simulink model "sampleModel2000"  (R2023a)
settings: Solver=VariableStepAuto  StartTime=0.0  StopTime=10.0  RelTol=1e-3
libraries: hdlsllib x4, simulink x2
settings Model: Creator=user1  LastModifiedBy=user1

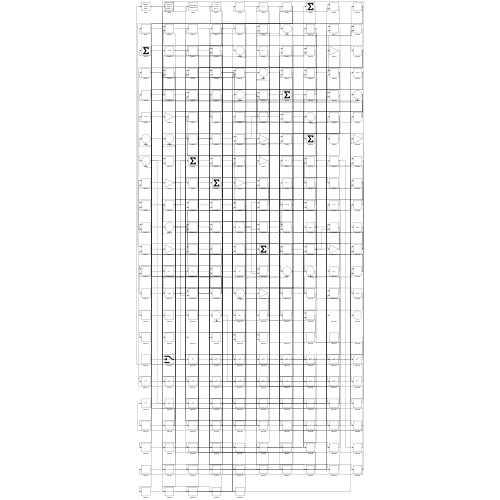
[thumbnail: Simulink's stored preview of the top-level diagram]
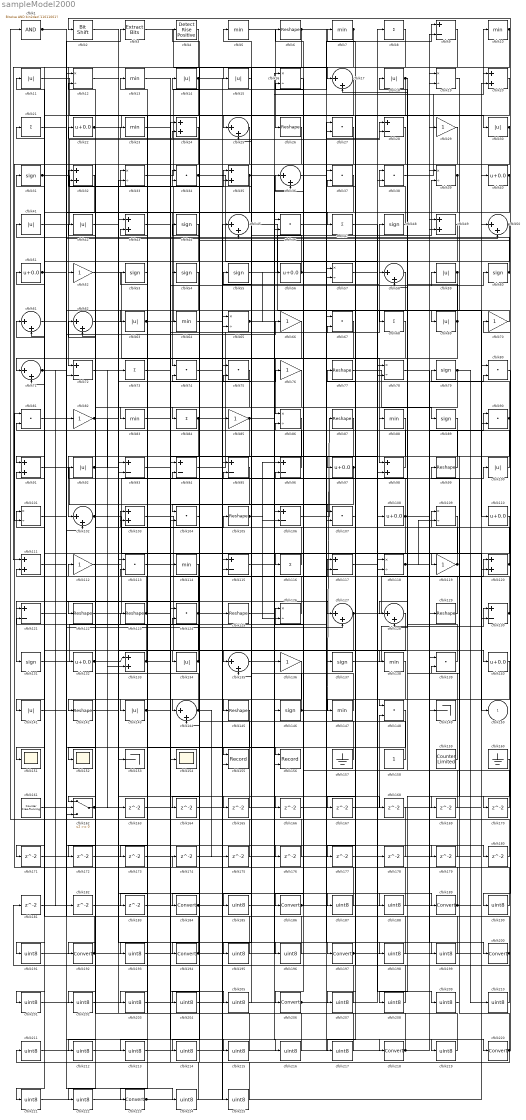
== system sampleModel2000 ==
  cfblk1 : simulink/Logic and Bit Operations/Bitwise Operator  logicop=AND  UseBitMask=on  BitMask=bin2dec('11011001')  BitMaskRealWorld=Stored Integer
      settings: LibrarySourceBlock=|
      | hdlsllib/Logic and Bit
      | Operations/Bitwise
      | Operator
  cfblk{5,7,10,13,23,64,83,88,114,138,147} (11 alike) : MinMax
  cfblk{11,14..15,18,30,41..42,59,63,69,92,100,134,141,143} (15 alike) : Abs  SaturateOnIntegerOverflow=off
  cfblk{12,16,19,33,39,57,65,78,86,101,109,118,126} (13 alike) : Product  Inputs=*/  RndMeth=Zero  SaturateOnIntegerOverflow=on
  cfblk{17,25,36,45,50,58,61..62,71,102,127..128,135,144} (14 alike) : Sum  Inputs=|++
  cfblk{20,24,32,35,43,49,91,98,103,111,120,133} (12 alike) : Sum
  cfblk{27,34,37..38,46,67,74..75,80..81,90,104,107,113,124,139,148} (17 alike) : DotProduct  OutDataTypeStr=Inherit: Inherit via internal rule
  cfblk{6,26,77,87,99,105,122..123,125,129,142,145} (12 alike) : Reshape
  cfblk{9,28,72,93..96,106,115,117,121,130} (12 alike) : Sum  Inputs=+-
  cfblk{22,40,51,56,97,108,110,132,140} (9 alike) : Bias  Bias=0.0  SaturateOnIntegerOverflow=off
  cfblk{29,52,66,70,76,82,85,112,119,136} (10 alike) : Gain
  cfblk{8,21,47,68,73,84,116} (7 alike) : Sum  Inputs=+
  cfblk{31,44,48,53..55,60,79,89,131,137,146} (12 alike) : Signum
  cfblk149 : Terminator
  cfblk151 : Scope
  cfblk152 : Scope
  cfblk153 : Terminator
  cfblk154 : Scope
  cfblk155 : Record  FileSettingsInternal="{\"entries\":[{\"content\":{\"excelSettings\":{\"content\":{},\"type\":\"Streamout.ExcelSettings\"}},\"type\":\"Streamout.FileSettingStorage\",\"uuid\":\"\"}],\"packageUris\":[\"http:\\/\\/schema.mathworks.com\\/mf0\\/streamout_blocks\\/R2020a\"],\"version\":\"1.0\"}"  Layout=[1 1]  SignalsInternal="{\"entries\":[{\"content\":{\"signals\":[{\"content\":{\"blockPath\":[],\"dimensions\":[1],\"domain\":\"\",\"lineColor\":\"#a2142f\",\"plots\":[1],\"port\":1,\"signalID\":5766,\"signalName\":\"XY Graph:1\"},\"type\":\"RecordBlkView.Signal\",\"uuid\":\"\"},{\"content\":{\"blockPath\":[],\"dimensions\":[1],\"domain\":\"\",\"lineColor\":\"#139fff\",\"plots\":[1],\"port\":2,\"signalID\":5769,\"signalName\":\"XY Graph:2\"},\"type\":\"RecordBlkView.Signal\",\"uuid\":\"\"}]},\"type\":\"RecordBlkView.InputSignals\",\"uuid\":\"\"}],\"packageUris\":[\"http:\\/\\/schema.mathworks.com\\/mf0\\/streamout_blocks\\/R2020a\"],\"version\":\"1.0\"}"  VisualizationBindings="{\"xyplotplugin\":{\"info\":[{\"series\":[{\"bindingParametersList\":[{\"parameter\":\"X-Axis\",\"signalID\":5766,\"signalName\":\"XY Graph:1\"},{\"parameter\":\"Y-Axis\",\"signalID\":5769,\"signalName\":\"XY Graph:2\"}],\"seriesID\":56463}],\"subplotID\":1}]}}"  CompatibilityTag=XY  st=-1
  cfblk156 : Record  FileSettingsInternal="{\"entries\":[{\"content\":{\"excelSettings\":{\"content\":{},\"type\":\"Streamout.ExcelSettings\"}},\"type\":\"Streamout.FileSettingStorage\",\"uuid\":\"\"}],\"packageUris\":[\"http:\\/\\/schema.mathworks.com\\/mf0\\/streamout_blocks\\/R2020a\"],\"version\":\"1.0\"}"  Layout=[1 1]  SignalsInternal="{\"entries\":[{\"content\":{\"signals\":[{\"content\":{\"blockPath\":[],\"dimensions\":[1],\"domain\":\"\",\"lineColor\":\"#a2142f\",\"plots\":[1],\"port\":1,\"signalID\":5774,\"signalName\":\"XY Graph:1\"},\"type\":\"RecordBlkView.Signal\",\"uuid\":\"\"},{\"content\":{\"blockPath\":[],\"dimensions\":[1],\"domain\":\"\",\"lineColor\":\"#139fff\",\"plots\":[1],\"port\":2,\"signalID\":5777,\"signalName\":\"XY Graph:2\"},\"type\":\"RecordBlkView.Signal\",\"uuid\":\"\"}]},\"type\":\"RecordBlkView.InputSignals\",\"uuid\":\"\"}],\"packageUris\":[\"http:\\/\\/schema.mathworks.com\\/mf0\\/streamout_blocks\\/R2020a\"],\"version\":\"1.0\"}"  VisualizationBindings="{\"xyplotplugin\":{\"info\":[{\"series\":[{\"bindingParametersList\":[{\"parameter\":\"X-Axis\",\"signalID\":5774,\"signalName\":\"XY Graph:1\"},{\"parameter\":\"Y-Axis\",\"signalID\":5777,\"signalName\":\"XY Graph:2\"}],\"seriesID\":7171}],\"subplotID\":1}]}}"  CompatibilityTag=XY  st=-1
  cfblk157 : Ground
  cfblk158 : Constant  SampleTime=-1
  cfblk159 : hdlsllib/Sources/Counter Limited  uplimit=7  tsamp=-1
  cfblk160 : Ground
  cfblk161 : hdlsllib/Sources/Counter Free-Running  NumBits=16  tsamp=-1
  cfblk162 : Switch  SaturateOnIntegerOverflow=off  InputSameDT=off
  cfblk{163..183} (21 alike) : Delay  SampleTime=1
  cfblk{184,186,189,192,194,197,200,206,218,220,223} (11 alike) : DataTypeConversion  SaturateOnIntegerOverflow=off  RndMeth=Floor
  cfblk{185,187..188,190..191,193,195..196,198..199,201..205,207..217,219,221..222,224..225} (31 alike) : DataTypeConversion  OutDataTypeStr=uint8  SaturateOnIntegerOverflow=off  RndMeth=Floor
  cfblk2 : hdlsllib/Logic and Bit Operations/Bit Shift  mode=Shift Left Logical  N=0
  cfblk3 : simulink/Logic and Bit Operations/Extract Bits  bitsToExtract=Upper half  numBits=8  bitIdxRange=[0 7]  outScalingMode=Preserve fixed-point scaling
      settings: LibrarySourceBlock=|
      | hdlsllib/Logic and Bit
      | Operations/Extract Bits
  cfblk4 : hdlsllib/Logic and Bit Operations/Detect Rise Positive  vinit=0  OutDataTypeStr=boolean
  cfblk150 : Outport  VectorParamsAs1DForOutWhenUnconnected=off
  wires:
  cfblk92/1 -> cfblk73/1, cfblk138/1
  cfblk22/1 -> cfblk25/1, cfblk188/1
  cfblk114/1 -> cfblk131/1
  cfblk105/1 -> cfblk96/1, cfblk106/2, cfblk126/2
  cfblk36/1 -> cfblk189/1
  cfblk162/1 -> cfblk165/1, cfblk166/1
  cfblk88/1 -> cfblk102/1
  cfblk84/1 -> cfblk180/1, cfblk202/1
  cfblk35/1 -> cfblk74/1, cfblk20/1, cfblk117/2
  cfblk77/1 -> cfblk89/1
  cfblk63/1 -> cfblk35/1, cfblk67/2
  cfblk4/1 -> cfblk111/1
  cfblk144/1 -> cfblk4/1, cfblk112/1, cfblk175/1
  cfblk147/1 -> cfblk55/1
  cfblk64/1 -> cfblk60/1
  cfblk54/1 -> cfblk83/1
  cfblk146/1 -> cfblk87/1, cfblk41/1
  cfblk134/1 -> cfblk11/1, cfblk121/2, cfblk123/1
  cfblk38/1 -> cfblk10/1
  cfblk42/1 -> cfblk153/1
  cfblk29/1 -> cfblk184/1
  cfblk124/1 -> cfblk101/1, cfblk58/1, cfblk162/1
  cfblk68/1 -> cfblk86/1
  cfblk16/1 -> cfblk186/1
  cfblk13/1 -> cfblk154/1
  cfblk9/1 -> cfblk14/1
  cfblk87/1 -> cfblk142/1
  cfblk27/1 -> cfblk116/1
  cfblk130/1 -> cfblk33/1, cfblk13/1
  cfblk103/1 -> cfblk135/1
  cfblk52/1 -> cfblk98/1
  cfblk136/1 -> cfblk192/1
  cfblk5/1 -> cfblk26/1
  cfblk102/1 -> cfblk46/1, cfblk150/1, cfblk133/2
  cfblk159/1 -> cfblk18/1
  cfblk98/1 -> cfblk86/2
  cfblk94/1 -> cfblk48/1
  cfblk50/1 -> cfblk122/1, cfblk104/1, cfblk128/1
  cfblk112/1 -> cfblk8/1
  cfblk18/1 -> cfblk88/1, cfblk217/1
  cfblk34/1 -> cfblk118/1, cfblk47/1, cfblk199/1
  cfblk121/1 -> cfblk127/1
  cfblk3/1 -> cfblk17/1
  cfblk59/1 -> cfblk156/1, cfblk162/3
  cfblk143/1 -> cfblk43/2, cfblk168/1
  cfblk110/1 -> cfblk137/1
  cfblk58/1 -> cfblk97/1
  cfblk132/1 -> cfblk133/1, cfblk124/2
  cfblk119/1 -> cfblk109/1, cfblk103/2
  cfblk7/1 -> cfblk72/1, cfblk191/1, cfblk214/1
  cfblk47/1 -> cfblk119/1
  cfblk62/1 -> cfblk125/1
  cfblk123/1 -> cfblk111/2, cfblk205/1
  cfblk100/1 -> cfblk44/1
  cfblk55/1 -> cfblk39/2
  cfblk116/1 -> cfblk5/1
  cfblk158/1 -> cfblk22/1
  cfblk61/1 -> cfblk82/1
  cfblk106/1 -> cfblk40/1
  cfblk122/1 -> cfblk105/1
  cfblk137/1 -> cfblk130/1
  cfblk73/1 -> cfblk59/1
  cfblk141/1 -> cfblk66/1
  cfblk40/1 -> cfblk141/1, cfblk162/2
  cfblk126/1 -> cfblk51/1
  cfblk23/1 -> cfblk218/1
  cfblk41/1 -> cfblk28/1
  cfblk128/1 -> cfblk151/1
  cfblk95/1 -> cfblk194/1
  cfblk45/1 -> cfblk110/1
  cfblk96/1 -> cfblk31/1
  cfblk157/1 -> cfblk126/1
  cfblk25/1 -> cfblk101/2
  cfblk82/1 -> cfblk76/1, cfblk163/1
  cfblk19/1 -> cfblk69/1
  cfblk11/1 -> cfblk93/2
  cfblk133/1 -> cfblk114/1, cfblk81/2, cfblk156/2, cfblk117/1
  cfblk60/1 -> cfblk21/1, cfblk34/2
  cfblk37/1 -> cfblk206/1
  cfblk74/1 -> cfblk85/1
  cfblk69/1 -> cfblk84/1, cfblk17/2
  cfblk120/1 -> cfblk2/1, cfblk77/1, cfblk32/1
  cfblk86/1 -> cfblk145/1
  cfblk30/1 -> cfblk72/2, cfblk63/1, cfblk144/2
  cfblk115/1 -> cfblk220/1
  cfblk76/1 -> cfblk134/1
  cfblk97/1 -> cfblk7/1, cfblk144/1
  cfblk70/1 -> cfblk68/1
  cfblk125/1 -> cfblk100/1
  cfblk91/1 -> cfblk146/1
  cfblk33/1 -> cfblk9/1
  cfblk90/1 -> cfblk79/1, cfblk128/2, cfblk169/1, cfblk170/1
  cfblk53/1 -> cfblk143/1
  cfblk81/1 -> cfblk3/1
  cfblk85/1 -> cfblk106/1, cfblk213/1
  cfblk43/1 -> cfblk98/2
  cfblk129/1 -> cfblk103/1
  cfblk72/1 -> cfblk107/1
  cfblk8/1 -> cfblk25/2
  cfblk39/1 -> cfblk52/1, cfblk177/1
  cfblk10/1 -> cfblk15/1, cfblk54/1
  cfblk2/1 -> cfblk30/1
  cfblk104/1 -> cfblk34/1
  cfblk140/1 -> cfblk148/1
  cfblk6/1 -> cfblk71/2, cfblk179/1
  cfblk17/1 -> cfblk91/1
  cfblk1/1 -> cfblk50/2, cfblk46/2
  cfblk108/1 -> cfblk90/1, cfblk42/1, cfblk171/1
  cfblk139/1 -> cfblk92/1
  cfblk31/1 -> cfblk35/2, cfblk224/1
  cfblk20/1 -> cfblk147/1
  cfblk145/1 -> cfblk155/1
  cfblk131/1 -> cfblk80/2
  cfblk99/1 -> cfblk53/1
  cfblk48/1 -> cfblk38/1
  cfblk78/1 -> cfblk200/1
  cfblk127/1 -> cfblk120/1, cfblk152/1
  cfblk44/1 -> cfblk121/1
  cfblk118/1 -> cfblk129/1, cfblk109/2
  cfblk93/1 -> cfblk64/1
  cfblk24/1 -> cfblk223/1
  cfblk161/1 -> cfblk132/1
  cfblk79/1 -> cfblk210/1, cfblk222/1
  cfblk51/1 -> cfblk127/2, cfblk71/1
  cfblk71/1 -> cfblk102/2, cfblk182/1
  cfblk101/1 -> cfblk155/2
  cfblk12/1 -> cfblk197/1
  cfblk65/1 -> cfblk140/1, cfblk56/1
  cfblk14/1 -> cfblk65/2, cfblk104/2, cfblk183/1
  cfblk56/1 -> cfblk28/2, cfblk32/2
  cfblk163/1 -> cfblk130/2
  cfblk66/1 -> cfblk164/1
  cfblk165/1 -> cfblk65/1
  cfblk166/1 -> cfblk148/2
  cfblk138/1 -> cfblk167/1
  cfblk167/1 -> cfblk50/1
  cfblk168/1 -> cfblk1/1
  cfblk169/1 -> cfblk96/2
  cfblk170/1 -> cfblk58/2
  cfblk171/1 -> cfblk107/2
  cfblk26/1 -> cfblk172/1
  cfblk172/1 -> cfblk33/2
  cfblk28/1 -> cfblk173/1
  cfblk173/1 -> cfblk118/2
  cfblk174/1 -> cfblk9/2
  cfblk175/1 -> cfblk93/1
  cfblk111/1 -> cfblk176/1
  cfblk176/1 -> cfblk61/1
  cfblk177/1 -> cfblk120/2
  cfblk117/1 -> cfblk178/1
  cfblk178/1 -> cfblk135/2
  cfblk179/1 -> cfblk94/2
  cfblk180/1 -> cfblk19/1
  cfblk181/1 -> cfblk38/2
  cfblk182/1 -> cfblk62/2
  cfblk183/1 -> cfblk45/2
  cfblk184/1 -> cfblk149/1, cfblk39/1
  cfblk15/1 -> cfblk185/1
  cfblk185/1 -> cfblk29/1
  cfblk186/1 -> cfblk6/1, cfblk80/1
  cfblk83/1 -> cfblk187/1
  cfblk187/1 -> cfblk16/1
  cfblk188/1 -> cfblk16/2
  cfblk189/1 -> cfblk174/1, cfblk81/1
  cfblk80/1 -> cfblk190/1
  cfblk190/1 -> cfblk36/1
  cfblk191/1 -> cfblk36/2
  cfblk192/1 -> cfblk91/2, cfblk61/2
  cfblk148/1 -> cfblk193/1
  cfblk193/1 -> cfblk136/1
  cfblk194/1 -> cfblk27/2, cfblk43/1
  cfblk109/1 -> cfblk195/1
  cfblk195/1 -> cfblk95/1
  cfblk142/1 -> cfblk196/1
  cfblk196/1 -> cfblk95/2
  cfblk197/1 -> cfblk20/2, cfblk19/2
  cfblk46/1 -> cfblk198/1
  cfblk198/1 -> cfblk12/1
  cfblk199/1 -> cfblk12/2
  cfblk200/1 -> cfblk181/1, cfblk27/1
  cfblk32/1 -> cfblk201/1
  cfblk201/1 -> cfblk78/1
  cfblk202/1 -> cfblk78/2
  cfblk75/1 -> cfblk203/1
  cfblk203/1 -> cfblk94/1
  cfblk89/1 -> cfblk204/1
  cfblk204/1 -> cfblk75/1
  cfblk205/1 -> cfblk75/2
  cfblk206/1 -> cfblk67/1, cfblk108/1
  cfblk107/1 -> cfblk207/1
  cfblk207/1 -> cfblk37/1
  cfblk160/1 -> cfblk208/1
  cfblk208/1 -> cfblk37/2
  cfblk57/1 -> cfblk209/1
  cfblk209/1 -> cfblk99/1
  cfblk210/1 -> cfblk57/1
  cfblk211/1 -> cfblk57/2
  cfblk49/1 -> cfblk212/1
  cfblk212/1 -> cfblk139/1
  cfblk213/1 -> cfblk49/1
  cfblk214/1 -> cfblk49/2
  cfblk113/1 -> cfblk215/1
  cfblk215/1 -> cfblk74/2
  cfblk21/1 -> cfblk216/1
  cfblk216/1 -> cfblk113/1
  cfblk217/1 -> cfblk113/2
  cfblk218/1 -> cfblk62/1, cfblk124/1
  cfblk135/1 -> cfblk219/1
  cfblk219/1 -> cfblk23/1
  cfblk220/1 -> cfblk211/1, cfblk139/2, cfblk70/1
  cfblk67/1 -> cfblk221/1
  cfblk221/1 -> cfblk115/1
  cfblk222/1 -> cfblk115/2
  cfblk223/1 -> cfblk90/2, cfblk45/1
  cfblk224/1 -> cfblk24/1
  cfblk164/1 -> cfblk225/1
  cfblk225/1 -> cfblk24/2
